simulink model "EDDobleP1"  (R2022b)
settings: Solver=VariableStepAuto  StartTime=0.0  StopTime=10  MaxStep=0.01  RelTol=1e-3
values from neighbouring files (symbols this model uses):
  g = 9.81    [parametrosEDDobleP.m]
  l1 = 0.3    [parametrosEDDobleP.m]
  l2 = 0.25    [parametrosEDDobleP.m]
  m1 = 0.2    [parametrosEDDobleP.m]
  m2 = 0.1    [parametrosEDDobleP.m]
settings Model: Creator=mluser  LastModifiedBy=mluser

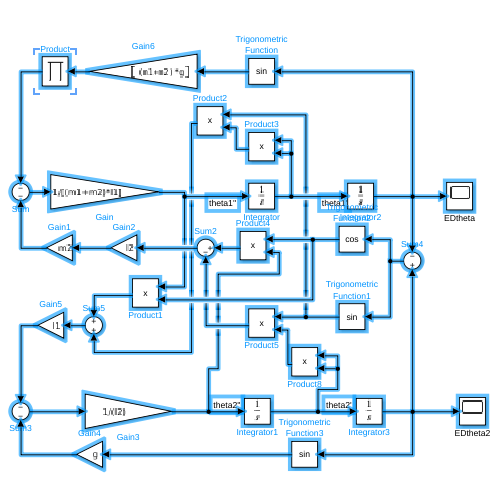
[thumbnail: Simulink's stored preview of the top-level diagram]
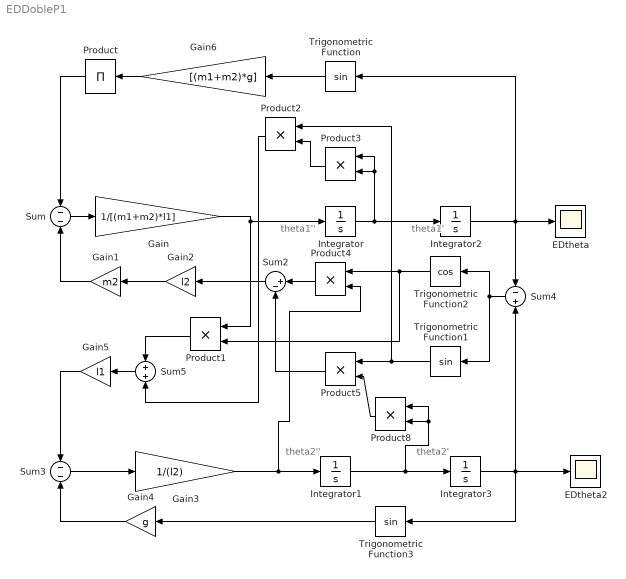
== system EDDobleP1 ==
  note: theta1''
  note: theta1'
  note: theta2'
  note: theta2''
  EDtheta : Scope
  EDtheta2 : Scope
  Gain : Gain  Gain=1/[(m1+m2)*l1]
  Gain1 : Gain  Gain=m2
  Gain2 : Gain  Gain=l2
  Gain3 : Gain  Gain=1/(l2)
  Gain4 : Gain  Gain=g
  Gain5 : Gain  Gain=l1
  Gain6 : Gain  Gain=[(m1+m2)*g]
  Integrator : Integrator
  Integrator1 : Integrator
  Integrator2 : Integrator
  Integrator3 : Integrator  InitialCondition=(35*pi)/180
  Product : Product  Inputs=1
  Product{1..5,8} (6 alike) : Product
  Sum : Sum  Inputs=--
  Sum2 : Sum  Inputs=|+-
  Sum3 : Sum  Inputs=--
  Sum4 : Sum  Inputs=-+
  Sum5 : Sum
  Trigonometric Function : Trigonometry
  Trigonometric Function1 : Trigonometry
  Trigonometric Function2 : Trigonometry  Operator=cos
  Trigonometric Function3 : Trigonometry
  wires:
  Gain/1 -> Product1/1, Integrator/1
  Sum/1 -> Gain/1
  Integrator/1 -> Integrator2/1, Product3/2, Product3/1
  Integrator2/1 -> Trigonometric Function/1, Sum4/1, EDtheta/1
  Product/1 -> Sum/1
  Integrator1/1 -> Product8/1, Product8/2, Integrator3/1
  Integrator3/1 -> Trigonometric Function3/1, EDtheta2/1, Sum4/2
  Sum3/1 -> Gain3/1
  Gain3/1 -> Product4/2, Integrator1/1
  Gain4/1 -> Sum3/2
  Trigonometric Function3/1 -> Gain4/1
  Sum4/1 -> Trigonometric Function1/1, Trigonometric Function2/1
  Product8/1 -> Product5/2
  Trigonometric Function1/1 -> Product5/1, Product2/1
  Trigonometric Function2/1 -> Product1/2, Product4/1
  Gain1/1 -> Sum/2
  Gain2/1 -> Gain1/1
  Sum2/1 -> Gain2/1
  Product4/1 -> Sum2/1
  Product5/1 -> Sum2/2
  Product1/1 -> Sum5/1
  Product2/1 -> Sum5/2
  Gain5/1 -> Sum3/1
  Sum5/1 -> Gain5/1
  Gain6/1 -> Product/1
  Product3/1 -> Product2/2
  Trigonometric Function/1 -> Gain6/1
